simulink model "IA331_lab9_1"  (R2023b)
settings: Solver=VariableStepAuto  StartTime=0.0  StopTime=10.0  RelTol=1e-3
model workspace (MAT data in the model file):
  lambda = 3
  max_prio = 10
  p_drop = 0.5
  service_time = 2
  u = 6
undefined symbols (not defined in the file): m, n
settings Model: Creator=jjake  LastModifiedBy=jjake

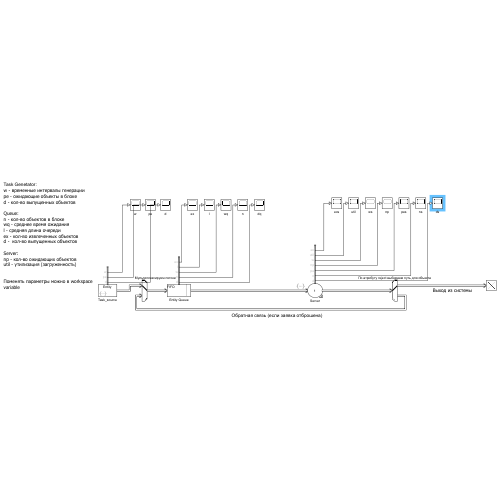
[thumbnail: Simulink's stored preview of the top-level diagram]
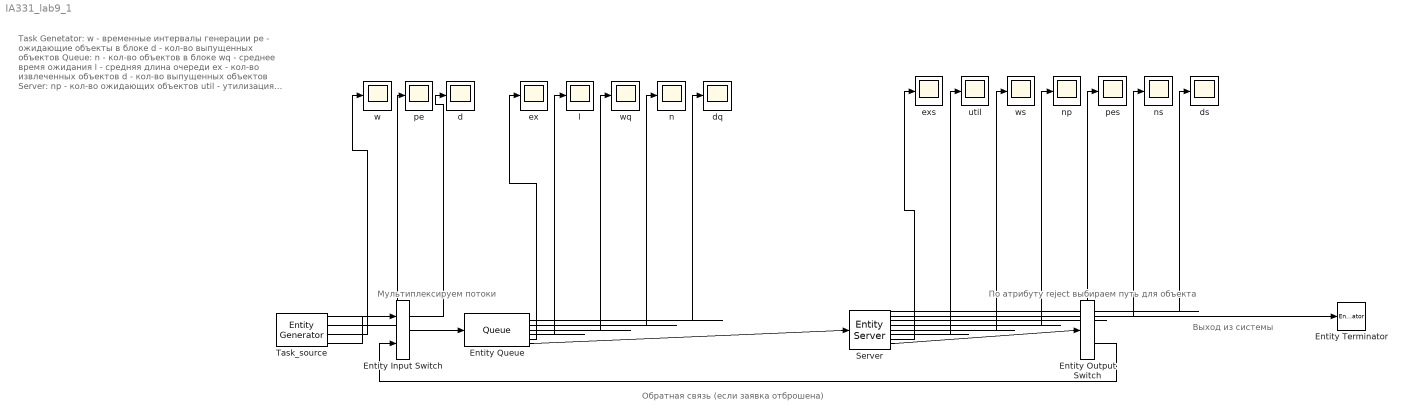
== system IA331_lab9_1 ==
  note: Мультиплексируем потоки
  note: По атрибуту reject выбираем путь для объекта
  note: Выход из системы
  note: Обратная связь (если заявка отброшена)
  note: Task Genetator:
      | w - временные интервалы генерации
      | pe - ожидающие объекты в блоке
      | d - кол-во выпущенных объектов
      |
      | Queue:
      | n - кол-во объектов в блоке
      | wq - среднее время ожидания
      | l - средняя длина очереди
      | ex - кол-во извлеченных объектов
      | d - кол-во выпущенных объектов
      |
      | Server:
      | np - кол-во ожидающих объектов
      | util - утилизация (загруженность)
      |
      | Поменять параметры можно в workspace
      | variable
  Entity Input Switch : EntityInputSwitch  InputPortMessageModes=m,m  OutputPortMessageModes=m  ActivePortSelection=Switch
  Entity Output Switch : EntityOutputSwitch  InputPortMessageModes=m  OutputPortMessageModes=m,m  SwitchingCriterion=From attribute  SwitchAttributeName=reject
  Entity Queue : Queue  InputPortMessageModes=m  OutputPortMessageModes=n,n,n,n,n,m  Capacity=6  NumberEntitiesDeparted=on  NumEntitiesExtracted=on  NumberEntitiesInBlock=on  AverageWait=on  AverageQueueLength=on
      settings: OutputPortMap=o0,o1,o2,o3,o7,o5
  Entity Terminator : EntityTerminator  InputPortMessageModes=m
  Server : EntityServer  InputPortMessageModes=m  OutputPortMessageModes=n,n,n,n,n,n,n,m,m  Capacity=1  ServiceTimeSource=MATLAB action  ServiceTimeAction=dt = exprnd(1/u);  EntryAction=|  PermitPreemptionBasedOnAttribute=on  SortingAttributeName=priority  NumberEntitiesDeparted=on  NumberEntitiesInBlock=on  PendingEntityPresentInBlock=on  NumberEntitiesPending=on  AverageWait=on  Utilization=on  NumEntitiesExtracted=on
      | r = rand();
      | 
      | if r < p_drop
      |     entity.reject = 1;
      | else
      |     entity.reject = 2;
      | end
      settings: OutputPortMap=o0,o1,o2,o3,o4,o5,o12,o9,o10
  Task_source : EntityGenerator  OutputPortMessageModes=n,n,n,m  TimeSource=MATLAB action  Period=1/lambda  IntergenerationTimeAction=dt = exprnd(1/lambda);  GenerateAction=|  AttributeName=priority|reject  AttributeInitialValue=1|1  NumberEntitiesDeparted=on  PendingEntityInBlock=on  AverageIntergenerationTime=on  EntityType=Structured  EntityTypeName=Entity  EntityPriority=1
      | id = 0;
      | id = id + 1;
      | Task_source.ID = id;
      settings: OutputPortMap=o0,o1,o2,o3
  d : Scope
  dq : Scope
  ds : Scope
  ex : Scope
  exs : Scope
  l : Scope
  n : Scope
  np : Scope
  ns : Scope
  pe : Scope
  pes : Scope
  util : Scope
  w : Scope
  wq : Scope
  ws : Scope
  wires:
  Task_source/3 -> w/1
  Task_source/2 -> pe/1
  Task_source/1 -> d/1
  Entity Queue/6 -> Server/1
  Server/7 -> exs/1
  Server/6 -> util/1
  Server/5 -> ws/1
  Server/4 -> np/1
  Server/3 -> pes/1
  Server/2 -> ns/1
  Server/1 -> ds/1
  Server/8 -> Entity Output Switch/1
  Entity Output Switch/1 -> Entity Terminator/1
  Entity Queue/5 -> ex/1
  Entity Queue/4 -> l/1
  Entity Queue/3 -> wq/1
  Entity Queue/2 -> n/1
  Entity Queue/1 -> dq/1
  Task_source/4 -> Entity Input Switch/1
  Entity Output Switch/2 -> Entity Input Switch/2
  Entity Input Switch/1 -> Entity Queue/1
